simulink model "lab2_PI_Tgz"  (Simulink 7.6)
settings: Solver=ode45  StartTime=0.0  StopTime=1000  RelTol=1e-3
values from neighbouring files (symbols this model uses):
  cpw = 4190    [lab2_sterowanie_Tgz.m]
  Cvg = cpw*row*Vg/4    (= 10265.5)    [lab2_sterowanie_Tgz.m]
  Cvw = cpp*rop*Vp    (= 23889.6)    [lab2_sterowanie_Tgz.m]
  dFg = 0    [lab2_sterowanie_Tgz.m]
  dQt = 0    [lab2_sterowanie_Tgz.m]
  dt = 100    [lab2_sterowanie_Tgz.m]
  dTwew_z = 2    [lab2_sterowanie_Tgz.m]
  dTzew = 0    [lab2_sterowanie_Tgz.m]
  Fg_0 = kg*(Tgsr_0-Twew_0)/(cpw*row*(Tgz_0-Tgp_0))    (= 0.000487068335687)    [lab2_sterowanie_Tgz.m]
  kg = Q_n/(Tgsr_n-Twew_n)    (= 400)    [lab2_sterowanie_Tgz.m]
  ki = .05    (= 0.05)    [lab2_sterowanie_Tgz.m]
  kp = 3.5    [lab2_sterowanie_Tgz.m]
  kw = (Q_n-Qt_n)/(Twew_n-Tzew_n)    (= 500)    [lab2_sterowanie_Tgz.m]
  Qt_0 = Qt_n    (= 0)    [lab2_sterowanie_Tgz.m]
  row = 980    [lab2_sterowanie_Tgz.m]
  Tgsr_0 = Tgp_0    (= 70)    [lab2_sterowanie_Tgz.m]
  Tr_0 = Tgz_0    (= 80)    [lab2_sterowanie_Tgz.m]
  Twew_0 = Twew_n    (= 20)    [lab2_sterowanie_Tgz.m]
  Twew_z0 = Twew_0    (= 20)    [lab2_sterowanie_Tgz.m]
  Tzew_0 = Tzew_n    (= -20)    [lab2_sterowanie_Tgz.m]
settings Model: Creator=LAB320-1537-User  LastModifiedBy=Tomek
settings DebuggingCC: FcnCallInpInsideContextMsg=Enable All
settings GRTTargetCC: CombineOutputUpdateFcns=on

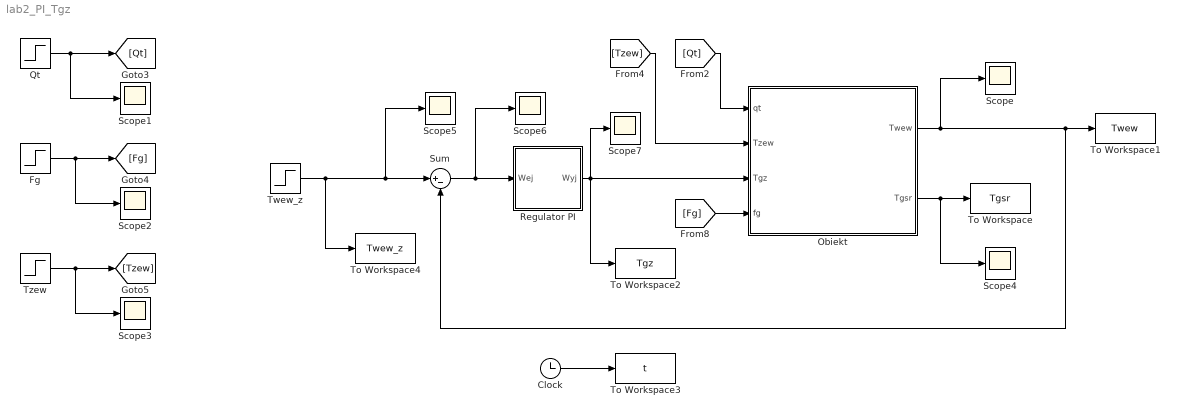
== system lab2_PI_Tgz ==
  Clock : Clock
      settings: Decimation=10
  Fg : Step  Time=dt  Before=Fg_0  After=Fg_0+dFg  SampleTime=0
  Obiekt : Subsystem  mask{Twew_0=Twew_0, Tgsr_0=Tgsr_0, kg=kg, kw=kw, Cvg=Cvg, Cvw=Cvw}
      mask prompts: Twew_0 "Temp. pocz. wewnatrz"; Tgsr_0 "Temp. pocz. grzejnika"; kg "Wsp. przewodzenia grzejnika"; kw "Wsp. przewodzenia scian"; Cvg "Pojemnosc cieplna grzejnika"; Cvw "Pojemnosc cieplna pomieszczenia"
  Qt : Step  Time=dt  Before=Qt_0  After=Qt_0+dQt  SampleTime=0
  Regulator PI : Subsystem  mask{kp=kp, ki=ki, Up=Tr_0}
      mask prompts: kp "Wzmocnienie reg. P"; ki "Wzmocnienie reg. I"; Up "Wartosc poczatkowa"
  Scope{,1..7} (8 alike) : Scope
      Scope settings: SaveName=ScopeData2
      Scope1 settings: SaveName=ScopeData3
      Scope3 settings: SaveName=ScopeData5
      Scope5 settings: SaveName=ScopeData4
      Scope6 settings: SaveName=ScopeData6
      Scope7 settings: SaveName=ScopeData7
  Sum : Sum  Inputs=|+-
  To Workspace : ToWorkspace  VariableName=Tgsr  SampleTime=-1  SaveFormat=Array
  To Workspace1 : ToWorkspace  VariableName=Twew  SampleTime=-1  SaveFormat=Array
  To Workspace2 : ToWorkspace  VariableName=Tgz  SampleTime=-1  SaveFormat=Array
  To Workspace3 : ToWorkspace  VariableName=t  SampleTime=-1  SaveFormat=Array
  To Workspace4 : ToWorkspace  VariableName=Twew_z  SampleTime=-1  SaveFormat=Array
  Twew_z : Step  Time=dt  Before=Twew_z0  After=Twew_z0+dTwew_z  SampleTime=0
  Tzew : Step  Time=dt  Before=Tzew_0  After=Tzew_0+dTzew  SampleTime=0
  wires:
  Qt/1 -> [Qt], Scope1/1
  Tzew/1 -> Scope3/1, [Tzew]
  [Qt] -> Obiekt/1(qt)
  Regulator PI/1(Wyj) -> Obiekt/3(Tgz), Scope7/1, To Workspace2/1
  [Fg] -> Obiekt/4(fg)
  Fg/1 -> Scope2/1, [Fg]
  Obiekt/1(Twew) -> Scope/1, To Workspace1/1, Sum/2
  Obiekt/2(Tgsr) -> To Workspace/1, Scope4/1
  [Tzew] -> Obiekt/2(Tzew)
  Sum/1 -> Regulator PI/1(Wej), Scope6/1
  Twew_z/1 -> Sum/1, Scope5/1, To Workspace4/1
  Clock/1 -> To Workspace3/1

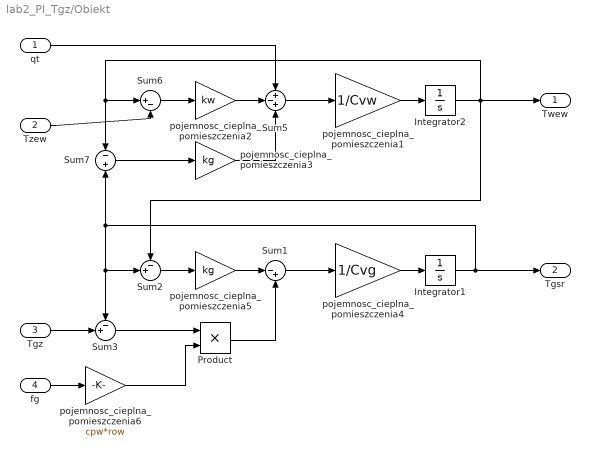
== system lab2_PI_Tgz/Obiekt ==
  qt : Inport
  Tzew : Inport  Port=2
  Tgz : Inport  Port=3
  fg : Inport  Port=4
  Integrator1 : Integrator  InitialCondition=Tgsr_0
  Integrator2 : Integrator  InitialCondition=Twew_0
  Product : Product  RndMeth=Zero
  Sum1 : Sum  Inputs=|-+
  Sum2 : Sum  Inputs=-+|
  Sum3 : Sum  Inputs=-+|
  Sum5 : Sum  Inputs=+-+
  Sum6 : Sum  Inputs=|+-
  Sum7 : Sum  Inputs=-|+
  pojemnosc_cieplna_pomieszczenia1 : Gain  Gain=1/Cvw
  pojemnosc_cieplna_pomieszczenia2 : Gain  Gain=kw
  pojemnosc_cieplna_pomieszczenia3 : Gain  Gain=kg
  pojemnosc_cieplna_pomieszczenia4 : Gain  Gain=1/Cvg
  pojemnosc_cieplna_pomieszczenia5 : Gain  Gain=kg
  pojemnosc_cieplna_pomieszczenia6 : Gain  Gain=cpw*row
  Twew : Outport
  Tgsr : Outport  Port=2
  wires:
  pojemnosc_cieplna_pomieszczenia1/1 -> Integrator2/1
  Integrator2/1 -> Sum2/1, Twew/1, Sum7/1, Sum6/1
  Sum5/1 -> pojemnosc_cieplna_pomieszczenia1/1
  pojemnosc_cieplna_pomieszczenia2/1 -> Sum5/2
  pojemnosc_cieplna_pomieszczenia3/1 -> Sum5/3
  Sum6/1 -> pojemnosc_cieplna_pomieszczenia2/1
  Sum7/1 -> pojemnosc_cieplna_pomieszczenia3/1
  pojemnosc_cieplna_pomieszczenia4/1 -> Integrator1/1
  Integrator1/1 -> Sum7/2, Sum2/2, Sum3/1, Tgsr/1
  Sum1/1 -> pojemnosc_cieplna_pomieszczenia4/1
  Sum2/1 -> pojemnosc_cieplna_pomieszczenia5/1
  pojemnosc_cieplna_pomieszczenia5/1 -> Sum1/1
  pojemnosc_cieplna_pomieszczenia6/1 -> Product/2
  Sum3/1 -> Product/1
  Product/1 -> Sum1/2
  qt/1 -> Sum5/1
  Tgz/1 -> Sum3/2
  fg/1 -> pojemnosc_cieplna_pomieszczenia6/1
  Tzew/1 -> Sum6/2

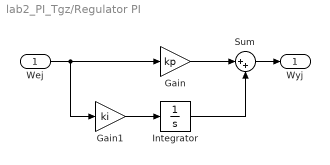
== system lab2_PI_Tgz/Regulator PI ==
  Wej : Inport
  Gain : Gain  Gain=kp
  Gain1 : Gain  Gain=ki
  Integrator : Integrator  InitialCondition=Up
  Sum : Sum  Inputs=|++
  Wyj : Outport
  wires:
  Gain/1 -> Sum/1
  Integrator/1 -> Sum/2
  Gain1/1 -> Integrator/1
  Wej/1 -> Gain/1, Gain1/1
  Sum/1 -> Wyj/1
